simulink model "dynamicmodel"  (Simulink 9.2)
settings: Solver=VariableStepAuto  StartTime=0.0  StopTime=4.0  RelTol=1e-3
undefined symbols (not defined in the file or in its folder): DiscIntNeverNeededParam, q0, q0_dot, Tc
settings Model: Creator=Harish  LastModifiedBy=Harish
settings DataIOCC: LimitDataPoints=off  SaveFormat=Dataset  SignalLoggingSaveFormat=Dataset  ReturnWorkspaceOutputs=on
settings OptimizationCC: LifeSpan=auto
settings DebuggingCC: UnderspecifiedInitializationDetection=Simplified  MergeDetectMultiDrivingBlocksExec=error  FcnCallInpInsideContextMsg=error  StateNameClashWarn=none  SFUnexpectedBacktrackingDiag=error  SFNoUnconditionalDefaultTransitionDiag=error  SFExecutionAtInitializationDiag=warning
settings HardwareCC: ProdBitPerPointer=64  ProdBitPerSizeT=64  ProdBitPerPtrDiffT=64  ProdLargestAtomicFloat=Float  ProdIntDivRoundTo=Zero  ProdEndianess=LittleEndian  ProdWordSize=64  ProdHWDeviceType=Intel->x86-64 (Windows64)
settings ModelReferenceCC: PropagateSignalLabelsOutOfModel=on
settings SFSimCC: SimUseLocalCustomCode=on
settings RTWCC: RTWUseLocalCustomCode=on
settings CodeAppCC: StateflowObjectComments=off
settings GRTTargetCC: TargetLangStandard=C99 (ISO)  GeneratePreprocessorConditionals=Use local settings  CombineOutputUpdateFcns=on  GRTInterface=off
settings ConfigComp: CovMetricSettings=dwe  CovHtmlReporting=off  CovSaveCumulativeToWorkspaceVar=off  CovSaveSingleToWorkspaceVar=off  CovExternalEMLEnable=on

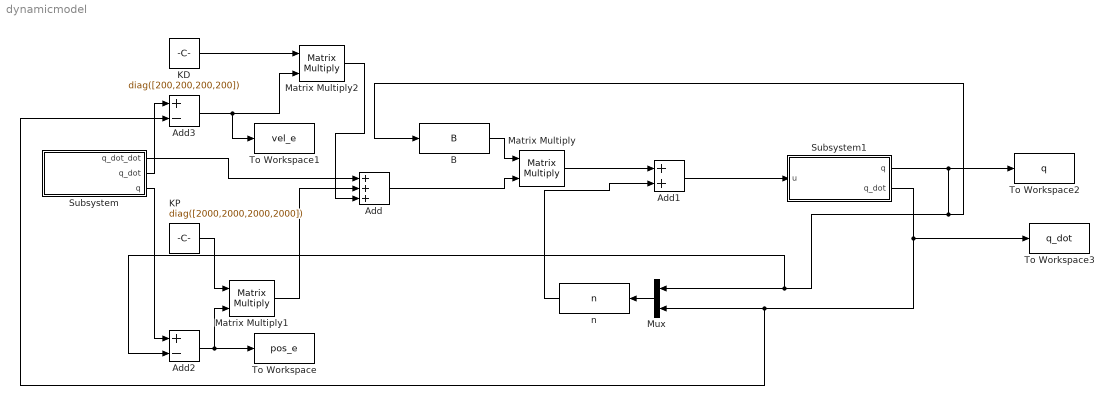
== system dynamicmodel ==
  Add : Sum  Inputs=+++
  Add1 : Sum
  Add2 : Sum  Inputs=+-
  Add3 : Sum  Inputs=+-
  B : MATLABFcn  MATLABFcn=B  Output1D=off
  KD : Constant  Value=diag([200,200,200,200])  VectorParams1D=off
  KP : Constant  Value=diag([2000,2000,2000,2000])  VectorParams1D=off
  Matrix Multiply : Product  Multiplication=Matrix(*)
  Matrix Multiply1 : Product  Multiplication=Matrix(*)
  Matrix Multiply2 : Product  Multiplication=Matrix(*)
  Mux : Mux  Inputs=2
  Subsystem : Subsystem
  Subsystem1 : Subsystem
  To Workspace : ToWorkspace  VariableName=pos_e  SampleTime=-1
  To Workspace1 : ToWorkspace  VariableName=vel_e  SampleTime=-1
  To Workspace2 : ToWorkspace  VariableName=q  SampleTime=-1
  To Workspace3 : ToWorkspace  VariableName=q_dot  SampleTime=-1
  n : MATLABFcn  MATLABFcn=n  Output1D=off
  wires:
  KD/1 -> Matrix Multiply2/1
  Subsystem/1(q_dot_dot) -> Add/1
  Add1/1 -> Subsystem1/1(u)
  Subsystem/3(q) -> Add2/1
  Matrix Multiply/1 -> Add1/1
  Matrix Multiply1/1 -> Add/2
  Add2/1 -> To Workspace/1, Matrix Multiply1/2
  KP/1 -> Matrix Multiply1/1
  Subsystem/2(q_dot) -> Add3/1
  Subsystem1/1(q) -> B/1, Add2/2, Mux/1, To Workspace2/1
  Subsystem1/2(q_dot) -> Mux/2, Add3/2, To Workspace3/1
  Matrix Multiply2/1 -> Add/3
  Add/1 -> Matrix Multiply/2
  Add3/1 -> To Workspace1/1, Matrix Multiply2/2
  B/1 -> Matrix Multiply/1
  n/1 -> Add1/2
  Mux/1 -> n/1

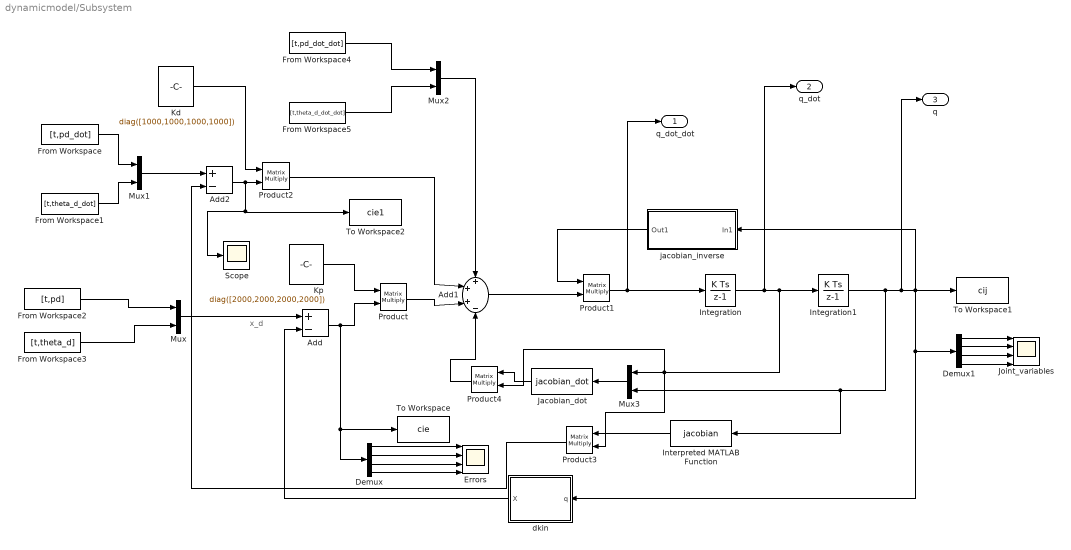
== system dynamicmodel/Subsystem ==
  note: x_d
  Add : Sum  Inputs=+-
  Add1 : Sum  Inputs=+++-
  Add2 : Sum  Inputs=+-
  Demux : Demux
  Demux1 : Demux
  Errors : Scope  NumInputPorts=4
  From Workspace : FromWorkspace  VariableName=[t,pd_dot]  SampleTime=0
  From Workspace1 : FromWorkspace  VariableName=[t,theta_d_dot]  SampleTime=0
  From Workspace2 : FromWorkspace  VariableName=[t,pd]  SampleTime=0
  From Workspace3 : FromWorkspace  VariableName=[t,theta_d]  SampleTime=0
  From Workspace4 : FromWorkspace  VariableName=[t,pd_dot_dot]  SampleTime=0
  From Workspace5 : FromWorkspace  VariableName=[t,theta_d_dot_dot]  SampleTime=0
  Integration : DiscreteIntegrator  InitialCondition=q0_dot  SampleTime=0.001  ICPrevOutput=DiscIntNeverNeededParam  ICPrevScaledInput=DiscIntNeverNeededParam
  Integration1 : DiscreteIntegrator  InitialCondition=q0  SampleTime=0.001  ICPrevOutput=DiscIntNeverNeededParam  ICPrevScaledInput=DiscIntNeverNeededParam
  Interpreted MATLAB Function : MATLABFcn  MATLABFcn=jacobian  Output1D=off
  Jacobian_dot : MATLABFcn  MATLABFcn=jacobian_dot  Output1D=off
  Joint_variables : Scope  NumInputPorts=4
  Kd : Constant  Value=diag([1000,1000,1000,1000])  VectorParams1D=off
  Kp : Constant  Value=diag([2000,2000,2000,2000])  VectorParams1D=off
  Mux{,1..3} (4 alike) : Mux  Inputs=2
  Product{,1..4} (5 alike) : Product  Multiplication=Matrix(*)
  Scope : Scope
  To Workspace : ToWorkspace  VariableName=cie  SaveFormat=Timeseries  SampleTime=-1
  To Workspace1 : ToWorkspace  VariableName=cij  SaveFormat=Timeseries  SampleTime=-1
  To Workspace2 : ToWorkspace  VariableName=cie1  SaveFormat=Timeseries  SampleTime=-1
  dkin : MATLAB Function  TreatAsAtomicUnit=on
  jacobian_inverse : Subsystem
  q_dot_dot : Outport
  q_dot : Outport  Port=2
  q : Outport  Port=3
  wires:
  dkin/1(X) -> Add/2
  Demux/3 -> Errors/3
  Add/1 -> To Workspace/1, Demux/1, Product/2
  Demux/2 -> Errors/2
  Demux1/3 -> Joint_variables/3
  From Workspace2/1 -> Mux/1
  Product/1 -> Add1/3
  From Workspace1/1 -> Mux1/2
  Kd/1 -> Product2/1
  Demux/4 -> Errors/4
  Mux3/1 -> Jacobian_dot/1
  Integration/1 -> q_dot/1, Product4/2, Product3/2, Mux3/1, Integration1/1
  Mux/1 -> Add/1
  Demux1/1 -> Joint_variables/1
  Demux/1 -> Errors/1
  Add1/1 -> Product1/2
  From Workspace3/1 -> Mux/2
  Integration1/1 -> Interpreted MATLAB Function/1, Mux3/2, q/1, jacobian_inverse/1(In1), Demux1/1, dkin/1(q), To Workspace1/1
  From Workspace4/1 -> Mux2/1
  Mux1/1 -> Add2/1
  jacobian_inverse/1(Out1) -> Product1/1
  Mux2/1 -> Add1/1
  Product3/1 -> Add2/2
  Product4/1 -> Add1/4
  Kp/1 -> Product/1
  Add2/1 -> Scope/1, To Workspace2/1, Product2/2
  Demux1/4 -> Joint_variables/4
  Jacobian_dot/1 -> Product4/1
  Demux1/2 -> Joint_variables/2
  Product2/1 -> Add1/2
  From Workspace5/1 -> Mux2/2
  From Workspace/1 -> Mux1/1
  Interpreted MATLAB Function/1 -> Product3/1
  Product1/1 -> q_dot_dot/1, Integration/1

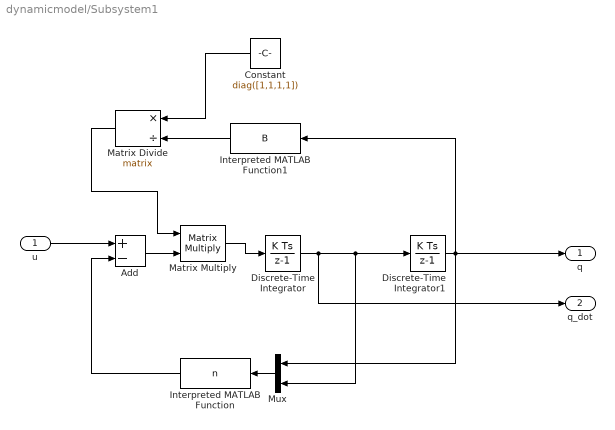
== system dynamicmodel/Subsystem1 ==
  u : Inport
  Add : Sum  Inputs=+-
  Constant : Constant  Value=diag([1,1,1,1])
  Discrete-Time Integrator : DiscreteIntegrator  InitialCondition=q0_dot  SampleTime=Tc  ICPrevOutput=DiscIntNeverNeededParam  ICPrevScaledInput=DiscIntNeverNeededParam
  Discrete-Time Integrator1 : DiscreteIntegrator  InitialCondition=q0  SampleTime=Tc  ICPrevOutput=DiscIntNeverNeededParam  ICPrevScaledInput=DiscIntNeverNeededParam
  Interpreted MATLAB Function : MATLABFcn  MATLABFcn=n  Output1D=off
  Interpreted MATLAB Function1 : MATLABFcn  MATLABFcn=B  Output1D=off
  Matrix Divide : Product  Inputs=*/  Multiplication=Matrix(*)
  Matrix Multiply : Product  Multiplication=Matrix(*)
  Mux : Mux  Inputs=2
  q : Outport
  q_dot : Outport  Port=2
  wires:
  Discrete-Time Integrator1/1 -> Mux/1, Interpreted MATLAB Function1/1, q/1
  Discrete-Time Integrator/1 -> q_dot/1, Mux/2, Discrete-Time Integrator1/1
  u/1 -> Add/1
  Interpreted MATLAB Function/1 -> Add/2
  Interpreted MATLAB Function1/1 -> Matrix Divide/2
  Constant/1 -> Matrix Divide/1
  Matrix Divide/1 -> Matrix Multiply/1
  Add/1 -> Matrix Multiply/2
  Matrix Multiply/1 -> Discrete-Time Integrator/1
  Mux/1 -> Interpreted MATLAB Function/1

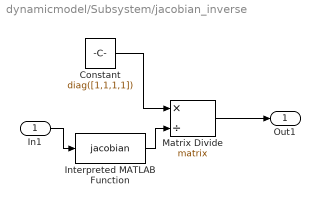
== system dynamicmodel/Subsystem/jacobian_inverse ==
  In1 : Inport
  Constant : Constant  Value=diag([1,1,1,1])
  Interpreted MATLAB Function : MATLABFcn  MATLABFcn=jacobian  Output1D=off
  Matrix Divide : Product  Inputs=*/  Multiplication=Matrix(*)
  Out1 : Outport
  wires:
  In1/1 -> Interpreted MATLAB Function/1
  Interpreted MATLAB Function/1 -> Matrix Divide/2
  Constant/1 -> Matrix Divide/1
  Matrix Divide/1 -> Out1/1

== matlab function Subsystem/dkin ==
  data: X output double; q input double
function X = direct_kin(q)
c1 = cos(q(1));
s1 = sin(q(1));
c2 = cos(q(2));
s2 = sin(q(2));
%d3 = c;
c12 = c1*c2-s1*s2;
s12 = s1*c2+s2*c1;
x = 0.5*c12+0.5*c1;
y = 0.5*s12+0.5*s1;
z = 1-q(3);
w = q(1)+q(2)+q(4);
%w = angle_rad - 2*pi*floor( (angle_rad+pi)/(2*pi) );
%w = wrapToPi(temp);
X = [x;y;z;w];
